simulink model "Full_Car_end_sem_Antiroll"  (R2023b)
settings: Solver=VariableStepAuto  StartTime=0.0  StopTime=20  FixedStep=0.00001  RelTol=1e-3
undefined symbols (not defined in the file): simscape, X, Y, Z
libraries: sm_lib x112, nesl_utility x70, fl_lib x23, sdl_lib x6, sharedtransform x4, simulink x2, simulink_extras x1
(part 6 of 6)

== system Full_Car_end_sem_Antiroll/Tire_RL/Tire_RL/Tire Visual ==
  Rigid Transform : sm_lib/Frames and Transforms/Rigid Transform  TranslationMethod=StandardAxis  TranslationStandardOffset=r0 - sectionHt/2  TranslationStandardOffsetUnits=m  TranslationStandardAxis=+Y  TranslationCartesianOffset=[0 0 0]  TranslationCartesianOffsetUnits=m  TranslationROffset=0  TranslationROffsetUnits=m  TranslationZOffset=0  TranslationZOffsetUnits=m  TranslationThetaOffset=0  TranslationThetaOffsetUnits=deg  RotationMethod=None  RotationAngleUnits=deg  RotationStandardAxis=+Z  RotationAngle=0.0  RotationArbitraryAxis=[0 0 1]  FollAlignAxisA=+X  BaseAlignAxisA=+Y  FollAlignAxisB=+Y  BaseAlignAxisB=+Z  RotationSequenceAxes=FollowerAxes  RotationSequence=XYX  RotationSequenceAngles=[0 0 0]  RotationSequenceAnglesUnits=deg  RotationMatrix=[1 0 0; 0 1 0; 0 0 1]  Quaternion=[1 0 0 0]
  Rigid Transform1 : sm_lib/Frames and Transforms/Rigid Transform  TranslationMethod=StandardAxis  TranslationStandardOffset=r0 - sectionHt/2  TranslationStandardOffsetUnits=m  TranslationStandardAxis=-Y  TranslationCartesianOffset=[0 0 0]  TranslationCartesianOffsetUnits=m  TranslationROffset=0  TranslationROffsetUnits=m  TranslationZOffset=0  TranslationZOffsetUnits=m  TranslationThetaOffset=0  TranslationThetaOffsetUnits=deg  RotationMethod=None  RotationAngleUnits=deg  RotationStandardAxis=+Z  RotationAngle=0.0  RotationArbitraryAxis=[0 0 1]  FollAlignAxisA=+X  BaseAlignAxisA=+Y  FollAlignAxisB=+Y  BaseAlignAxisB=+Z  RotationSequenceAxes=FollowerAxes  RotationSequence=XYX  RotationSequenceAngles=[0 0 0]  RotationSequenceAnglesUnits=deg  RotationMatrix=[1 0 0; 0 1 0; 0 0 1]  Quaternion=[1 0 0 0]
  Rigid Transform2 : sm_lib/Frames and Transforms/Rigid Transform  TranslationMethod=StandardAxis  TranslationStandardOffset=lr_val*(rimWidth/2-0.01)  TranslationStandardOffsetUnits=m  TranslationStandardAxis=+Z  TranslationCartesianOffset=[0 0 0]  TranslationCartesianOffsetUnits=m  TranslationROffset=0  TranslationROffsetUnits=m  TranslationZOffset=0  TranslationZOffsetUnits=m  TranslationThetaOffset=0  TranslationThetaOffsetUnits=deg  RotationMethod=None  RotationAngleUnits=deg  RotationStandardAxis=+Z  RotationAngle=0.0  RotationArbitraryAxis=[0 0 1]  FollAlignAxisA=+X  BaseAlignAxisA=+Y  FollAlignAxisB=+Y  BaseAlignAxisB=+Z  RotationSequenceAxes=FollowerAxes  RotationSequence=XYX  RotationSequenceAngles=[0 0 0]  RotationSequenceAnglesUnits=deg  RotationMatrix=[1 0 0; 0 1 0; 0 0 1]  Quaternion=[1 0 0 0]
  Rim : sm_lib/Body Elements/Extruded Solid  GraphicAmbientColor=[0.15 0.15 0.15 1.0]  BasedOnType=Density  CenterOfMass=[0 0 0]  CenterOfMassUnits=m  GraphicDiffuseColor=pulley_clr  ExportConvexHullGeometry=off  ExtrusionCrossSection=[x_rim',y_rim']  ExtrusionCrossSectionUnits=m  Density=0.001  DensityUnits=kg/m^3  DoExposeReferenceFrame=on  GraphicEmissiveColor=[0.0 0.0 0.0 1.0]  ExportEntireGeometry=off  ExtrusionLength=rimWidth  ExtrusionLengthUnits=m  ExtrusionType=General  SerializedFrames=<Frames/>  MarkerShape=Sphere  MarkerSize=10  GraphicType=FromGeometry  InertiaType=CalculateFromGeometry  Mass=1  MassUnits=kg  MomentsOfInertia=[1 1 1]  MomentsOfInertiaUnits=kg*m^2  PolygonNumSides=3  GraphicOpacity=pulley_opc  PolygonOuterRadius=1  PolygonOuterRadiusUnits=m  ProductsOfInertia=[0 0 0]  ProductsOfInertiaUnits=kg*m^2  GraphicShininess=75  GraphicSpecularColor=[0.5 0.5 0.5 1.0]  GraphicVisPropType=SimpleVisualProperties
  Rim design : sm_lib/Body Elements/Extruded Solid  GraphicAmbientColor=[0.15 0.15 0.15 1.0]  BasedOnType=Density  CenterOfMass=[0 0 0]  CenterOfMassUnits=m  GraphicDiffuseColor=pulley_clr  ExportConvexHullGeometry=off  ExtrusionCrossSection=[X,Y]  ExtrusionCrossSectionUnits=m  Density=0.001  DensityUnits=kg/m^3  DoExposeReferenceFrame=on  GraphicEmissiveColor=[0.0 0.0 0.0 1.0]  ExportEntireGeometry=off  ExtrusionLength=0.02  ExtrusionLengthUnits=m  ExtrusionType=General  SerializedFrames=<Frames/>  MarkerShape=Sphere  MarkerSize=10  GraphicType=FromGeometry  InertiaType=CalculateFromGeometry  Mass=1  MassUnits=kg  MomentsOfInertia=[1 1 1]  MomentsOfInertiaUnits=kg*m^2  PolygonNumSides=3  GraphicOpacity=pulley_opc  PolygonOuterRadius=1  PolygonOuterRadiusUnits=m  ProductsOfInertia=[0 0 0]  ProductsOfInertiaUnits=kg*m^2  GraphicShininess=75  GraphicSpecularColor=[0.5 0.5 0.5 1.0]  GraphicVisPropType=SimpleVisualProperties
  Tire : sm_lib/Body Elements/Extruded Solid  GraphicAmbientColor=[0.15 0.15 0.15 1.0]  BasedOnType=Density  CenterOfMass=[0 0 0]  CenterOfMassUnits=m  GraphicDiffuseColor=box_color  ExportConvexHullGeometry=off  ExtrusionCrossSection=[x_tire',y_tire']  ExtrusionCrossSectionUnits=m  Density=0.001  DensityUnits=kg/m^3  DoExposeReferenceFrame=on  GraphicEmissiveColor=[0.0 0.0 0.0 1.0]  ExportEntireGeometry=off  ExtrusionLength=rimWidth  ExtrusionLengthUnits=m  ExtrusionType=General  SerializedFrames=<Frames/>  MarkerShape=Sphere  MarkerSize=10  GraphicType=FromGeometry  InertiaType=CalculateFromGeometry  Mass=1  MassUnits=kg  MomentsOfInertia=[1 1 1]  MomentsOfInertiaUnits=kg*m^2  PolygonNumSides=3  GraphicOpacity=box_opc  PolygonOuterRadius=1  PolygonOuterRadiusUnits=m  ProductsOfInertia=[0 0 0]  ProductsOfInertiaUnits=kg*m^2  GraphicShininess=75  GraphicSpecularColor=[0.5 0.5 0.5 1.0]  GraphicVisPropType=SimpleVisualProperties
  C : PMIOPort  Side=Left
  connections:
  Rim design/RConn1 -- Rigid Transform2/RConn1
  Rigid Transform/RConn1 -- Rim/RConn1 -- Rigid Transform2/LConn1
  Rigid Transform/LConn1 -- Rigid Transform1/RConn1
  Rigid Transform1/LConn1 -- Tire/RConn1 -- C/RConn1

== system Full_Car_end_sem_Antiroll/Tire_RR/Tire_RR/Tire Visual ==
  Rigid Transform : sm_lib/Frames and Transforms/Rigid Transform  TranslationMethod=StandardAxis  TranslationStandardOffset=r0 - sectionHt/2  TranslationStandardOffsetUnits=m  TranslationStandardAxis=+Y  TranslationCartesianOffset=[0 0 0]  TranslationCartesianOffsetUnits=m  TranslationROffset=0  TranslationROffsetUnits=m  TranslationZOffset=0  TranslationZOffsetUnits=m  TranslationThetaOffset=0  TranslationThetaOffsetUnits=deg  RotationMethod=None  RotationAngleUnits=deg  RotationStandardAxis=+Z  RotationAngle=0.0  RotationArbitraryAxis=[0 0 1]  FollAlignAxisA=+X  BaseAlignAxisA=+Y  FollAlignAxisB=+Y  BaseAlignAxisB=+Z  RotationSequenceAxes=FollowerAxes  RotationSequence=XYX  RotationSequenceAngles=[0 0 0]  RotationSequenceAnglesUnits=deg  RotationMatrix=[1 0 0; 0 1 0; 0 0 1]  Quaternion=[1 0 0 0]
  Rigid Transform1 : sm_lib/Frames and Transforms/Rigid Transform  TranslationMethod=StandardAxis  TranslationStandardOffset=r0 - sectionHt/2  TranslationStandardOffsetUnits=m  TranslationStandardAxis=-Y  TranslationCartesianOffset=[0 0 0]  TranslationCartesianOffsetUnits=m  TranslationROffset=0  TranslationROffsetUnits=m  TranslationZOffset=0  TranslationZOffsetUnits=m  TranslationThetaOffset=0  TranslationThetaOffsetUnits=deg  RotationMethod=None  RotationAngleUnits=deg  RotationStandardAxis=+Z  RotationAngle=0.0  RotationArbitraryAxis=[0 0 1]  FollAlignAxisA=+X  BaseAlignAxisA=+Y  FollAlignAxisB=+Y  BaseAlignAxisB=+Z  RotationSequenceAxes=FollowerAxes  RotationSequence=XYX  RotationSequenceAngles=[0 0 0]  RotationSequenceAnglesUnits=deg  RotationMatrix=[1 0 0; 0 1 0; 0 0 1]  Quaternion=[1 0 0 0]
  Rigid Transform2 : sm_lib/Frames and Transforms/Rigid Transform  TranslationMethod=StandardAxis  TranslationStandardOffset=lr_val*(rimWidth/2-0.01)  TranslationStandardOffsetUnits=m  TranslationStandardAxis=+Z  TranslationCartesianOffset=[0 0 0]  TranslationCartesianOffsetUnits=m  TranslationROffset=0  TranslationROffsetUnits=m  TranslationZOffset=0  TranslationZOffsetUnits=m  TranslationThetaOffset=0  TranslationThetaOffsetUnits=deg  RotationMethod=None  RotationAngleUnits=deg  RotationStandardAxis=+Z  RotationAngle=0.0  RotationArbitraryAxis=[0 0 1]  FollAlignAxisA=+X  BaseAlignAxisA=+Y  FollAlignAxisB=+Y  BaseAlignAxisB=+Z  RotationSequenceAxes=FollowerAxes  RotationSequence=XYX  RotationSequenceAngles=[0 0 0]  RotationSequenceAnglesUnits=deg  RotationMatrix=[1 0 0; 0 1 0; 0 0 1]  Quaternion=[1 0 0 0]
  Rim : sm_lib/Body Elements/Extruded Solid  GraphicAmbientColor=[0.15 0.15 0.15 1.0]  BasedOnType=Density  CenterOfMass=[0 0 0]  CenterOfMassUnits=m  GraphicDiffuseColor=pulley_clr  ExportConvexHullGeometry=off  ExtrusionCrossSection=[x_rim',y_rim']  ExtrusionCrossSectionUnits=m  Density=0.001  DensityUnits=kg/m^3  DoExposeReferenceFrame=on  GraphicEmissiveColor=[0.0 0.0 0.0 1.0]  ExportEntireGeometry=off  ExtrusionLength=rimWidth  ExtrusionLengthUnits=m  ExtrusionType=General  SerializedFrames=<Frames/>  MarkerShape=Sphere  MarkerSize=10  GraphicType=FromGeometry  InertiaType=CalculateFromGeometry  Mass=1  MassUnits=kg  MomentsOfInertia=[1 1 1]  MomentsOfInertiaUnits=kg*m^2  PolygonNumSides=3  GraphicOpacity=pulley_opc  PolygonOuterRadius=1  PolygonOuterRadiusUnits=m  ProductsOfInertia=[0 0 0]  ProductsOfInertiaUnits=kg*m^2  GraphicShininess=75  GraphicSpecularColor=[0.5 0.5 0.5 1.0]  GraphicVisPropType=SimpleVisualProperties
  Rim design : sm_lib/Body Elements/Extruded Solid  GraphicAmbientColor=[0.15 0.15 0.15 1.0]  BasedOnType=Density  CenterOfMass=[0 0 0]  CenterOfMassUnits=m  GraphicDiffuseColor=pulley_clr  ExportConvexHullGeometry=off  ExtrusionCrossSection=[X,Y]  ExtrusionCrossSectionUnits=m  Density=0.001  DensityUnits=kg/m^3  DoExposeReferenceFrame=on  GraphicEmissiveColor=[0.0 0.0 0.0 1.0]  ExportEntireGeometry=off  ExtrusionLength=0.02  ExtrusionLengthUnits=m  ExtrusionType=General  SerializedFrames=<Frames/>  MarkerShape=Sphere  MarkerSize=10  GraphicType=FromGeometry  InertiaType=CalculateFromGeometry  Mass=1  MassUnits=kg  MomentsOfInertia=[1 1 1]  MomentsOfInertiaUnits=kg*m^2  PolygonNumSides=3  GraphicOpacity=pulley_opc  PolygonOuterRadius=1  PolygonOuterRadiusUnits=m  ProductsOfInertia=[0 0 0]  ProductsOfInertiaUnits=kg*m^2  GraphicShininess=75  GraphicSpecularColor=[0.5 0.5 0.5 1.0]  GraphicVisPropType=SimpleVisualProperties
  Tire : sm_lib/Body Elements/Extruded Solid  GraphicAmbientColor=[0.15 0.15 0.15 1.0]  BasedOnType=Density  CenterOfMass=[0 0 0]  CenterOfMassUnits=m  GraphicDiffuseColor=box_color  ExportConvexHullGeometry=off  ExtrusionCrossSection=[x_tire',y_tire']  ExtrusionCrossSectionUnits=m  Density=0.001  DensityUnits=kg/m^3  DoExposeReferenceFrame=on  GraphicEmissiveColor=[0.0 0.0 0.0 1.0]  ExportEntireGeometry=off  ExtrusionLength=rimWidth  ExtrusionLengthUnits=m  ExtrusionType=General  SerializedFrames=<Frames/>  MarkerShape=Sphere  MarkerSize=10  GraphicType=FromGeometry  InertiaType=CalculateFromGeometry  Mass=1  MassUnits=kg  MomentsOfInertia=[1 1 1]  MomentsOfInertiaUnits=kg*m^2  PolygonNumSides=3  GraphicOpacity=box_opc  PolygonOuterRadius=1  PolygonOuterRadiusUnits=m  ProductsOfInertia=[0 0 0]  ProductsOfInertiaUnits=kg*m^2  GraphicShininess=75  GraphicSpecularColor=[0.5 0.5 0.5 1.0]  GraphicVisPropType=SimpleVisualProperties
  C : PMIOPort  Side=Left
  connections:
  C/RConn1 -- Tire/RConn1 -- Rigid Transform1/LConn1
  Rigid Transform/LConn1 -- Rigid Transform1/RConn1
  Rigid Transform2/LConn1 -- Rim/RConn1 -- Rigid Transform/RConn1
  Rim design/RConn1 -- Rigid Transform2/RConn1

== system Full_Car_end_sem_Antiroll/6 DOF/Tx Sensor/non rotating follower - vehicle frame/AngAccl1 ==
  bx : Inport
  by : Inport  Port=2
  bz : Inport  Port=3
  bus creator4 : BusCreator  Inputs=3
  AngAccl : Outport
  wires:
  bx/1 -> bus creator4/1  "bx"
  by/1 -> bus creator4/2  "by"
  bz/1 -> bus creator4/3  "bz"
  bus creator4/1 -> AngAccl/1  "AngAcclVehFrame"

== system Full_Car_end_sem_Antiroll/6 DOF/Tx Sensor/non rotating follower - vehicle frame/Angvel1 ==
  wx : Inport
  wy : Inport  Port=2
  wz : Inport  Port=3
  bus creator4 : BusCreator  Inputs=3
  AngVel : Outport
  wires:
  bus creator4/1 -> AngVel/1  "AngVelVehFrame"
  wz/1 -> bus creator4/3  "wz"
  wy/1 -> bus creator4/2  "wy"
  wx/1 -> bus creator4/1  "wx"

== system Full_Car_end_sem_Antiroll/6 DOF/Tx Sensor/non rotating follower - vehicle frame/LinAccl1 ==
  ax : Inport
  ay : Inport  Port=2
  az : Inport  Port=3
  bus creator2 : BusCreator  Inputs=3
  LinAccl : Outport
  wires:
  bus creator2/1 -> LinAccl/1  "LinAcclVehFrame"
  az/1 -> bus creator2/3  "az"
  ax/1 -> bus creator2/1  "ax"
  ay/1 -> bus creator2/2  "ay"

== system Full_Car_end_sem_Antiroll/6 DOF/Tx Sensor/non rotating follower - vehicle frame/LinPos1 ==
  px : Inport
  py : Inport  Port=2
  pz : Inport  Port=3
  bus creator : BusCreator  Inputs=3
  LinPos : Outport
  wires:
  bus creator/1 -> LinPos/1  "LinPosVehFrame"
  px/1 -> bus creator/1  "px"
  pz/1 -> bus creator/3  "pz"
  py/1 -> bus creator/2  "py"

== system Full_Car_end_sem_Antiroll/6 DOF/Tx Sensor/non rotating follower - vehicle frame/LinVel1 ==
  vx : Inport
  vy : Inport  Port=2
  vz : Inport  Port=3
  bus creator1 : BusCreator  Inputs=3
  LinVel : Outport
  wires:
  vz/1 -> bus creator1/3  "vz"
  vy/1 -> bus creator1/2  "vy"
  vx/1 -> bus creator1/1  "vx"
  bus creator1/1 -> LinVel/1  "LinVelVehFrame"

== system Full_Car_end_sem_Antiroll/6 DOF/Tx Sensor/non rotating follower - vehicle frame/quaternion to angle1 ==
  q : Inport
  Quaternions to Rotation Angles : sharedtransform/Quaternions to Rotation Angles  rotationOrder=ZYX  aMode=aMode
  Selector : Selector  InputPortWidth=3  IndexOptions=Index vector (dialog)  Indices=3  OutputSizes=1
  Selector1 : Selector  InputPortWidth=3  IndexOptions=Index vector (dialog)  Indices=2  OutputSizes=1
  Selector2 : Selector  InputPortWidth=3  IndexOptions=Index vector (dialog)  Indices=1  OutputSizes=1
  bus creator3 : BusCreator  Inputs=3
  Ang : Outport
  wires:
  Quaternions to Rotation Angles/1 -> Selector1/1, Selector2/1, Selector/1
  Selector1/1 -> bus creator3/2  "ry"
  bus creator3/1 -> Ang/1  "AngVehFrame"
  Selector2/1 -> bus creator3/3  "rz"
  Selector/1 -> bus creator3/1  "rx"
  q/1 -> Quaternions to Rotation Angles/1

== system Full_Car_end_sem_Antiroll/6 DOF/Tx Sensor/world frame/AngAccl ==
  bx : Inport
  by : Inport  Port=2
  bz : Inport  Port=3
  bus creator4 : BusCreator  Inputs=3
  AngAccl : Outport
  wires:
  bus creator4/1 -> AngAccl/1  "AngAccl"
  bz/1 -> bus creator4/3  "bz"
  by/1 -> bus creator4/2  "by"
  bx/1 -> bus creator4/1  "bx"

== system Full_Car_end_sem_Antiroll/6 DOF/Tx Sensor/world frame/Angvel ==
  wx : Inport
  wy : Inport  Port=2
  wz : Inport  Port=3
  bus creator4 : BusCreator  Inputs=3
  AngVel : Outport
  wires:
  wx/1 -> bus creator4/1  "wx"
  wy/1 -> bus creator4/2  "wy"
  wz/1 -> bus creator4/3  "wz"
  bus creator4/1 -> AngVel/1  "AngVel"

== system Full_Car_end_sem_Antiroll/6 DOF/Tx Sensor/world frame/LinAccl ==
  ax : Inport
  ay : Inport  Port=2
  az : Inport  Port=3
  bus creator2 : BusCreator  Inputs=3
  LinAccl : Outport
  wires:
  ay/1 -> bus creator2/2  "ay"
  ax/1 -> bus creator2/1  "ax"
  az/1 -> bus creator2/3  "az"
  bus creator2/1 -> LinAccl/1  "LinAccl"

== system Full_Car_end_sem_Antiroll/6 DOF/Tx Sensor/world frame/LinPos ==
  px : Inport
  py : Inport  Port=2
  pz : Inport  Port=3
  bus creator : BusCreator  Inputs=3
  LinPos : Outport
  wires:
  py/1 -> bus creator/2  "py"
  pz/1 -> bus creator/3  "pz"
  px/1 -> bus creator/1  "px"
  bus creator/1 -> LinPos/1  "LinPos"

== system Full_Car_end_sem_Antiroll/6 DOF/Tx Sensor/world frame/LinVel ==
  vx : Inport
  vy : Inport  Port=2
  vz : Inport  Port=3
  bus creator1 : BusCreator  Inputs=3
  LinVel : Outport
  wires:
  bus creator1/1 -> LinVel/1  "LinVel"
  vx/1 -> bus creator1/1  "vx"
  vy/1 -> bus creator1/2  "vy"
  vz/1 -> bus creator1/3  "vz"

== system Full_Car_end_sem_Antiroll/6 DOF/Tx Sensor/world frame/quaternion to angle ==
  q : Inport
  Quaternions to Rotation Angles : sharedtransform/Quaternions to Rotation Angles  rotationOrder=ZYX  aMode=aMode
  Selector : Selector  InputPortWidth=3  IndexOptions=Index vector (dialog)  Indices=3  OutputSizes=1
  Selector1 : Selector  InputPortWidth=3  IndexOptions=Index vector (dialog)  Indices=2  OutputSizes=1
  Selector2 : Selector  InputPortWidth=3  IndexOptions=Index vector (dialog)  Indices=1  OutputSizes=1
  bus creator3 : BusCreator  Inputs=3
  Ang : Outport
  wires:
  q/1 -> Quaternions to Rotation Angles/1
  Selector/1 -> bus creator3/1  "rx"
  Selector2/1 -> bus creator3/3  "rz"
  bus creator3/1 -> Ang/1  "Ang"
  Selector1/1 -> bus creator3/2  "ry"
  Quaternions to Rotation Angles/1 -> Selector/1, Selector2/1, Selector1/1

== system Full_Car_end_sem_Antiroll/6DOF CG/Tx Sensor/non rotating follower - vehicle frame/AngAccl1 ==
  bx : Inport
  by : Inport  Port=2
  bz : Inport  Port=3
  bus creator4 : BusCreator  Inputs=3
  AngAccl : Outport
  wires:
  bx/1 -> bus creator4/1  "bx"
  by/1 -> bus creator4/2  "by"
  bz/1 -> bus creator4/3  "bz"
  bus creator4/1 -> AngAccl/1  "AngAcclVehFrame"

== system Full_Car_end_sem_Antiroll/6DOF CG/Tx Sensor/non rotating follower - vehicle frame/Angvel1 ==
  wx : Inport
  wy : Inport  Port=2
  wz : Inport  Port=3
  bus creator4 : BusCreator  Inputs=3
  AngVel : Outport
  wires:
  bus creator4/1 -> AngVel/1  "AngVelVehFrame"
  wz/1 -> bus creator4/3  "wz"
  wy/1 -> bus creator4/2  "wy"
  wx/1 -> bus creator4/1  "wx"

== system Full_Car_end_sem_Antiroll/6DOF CG/Tx Sensor/non rotating follower - vehicle frame/LinAccl1 ==
  ax : Inport
  ay : Inport  Port=2
  az : Inport  Port=3
  bus creator2 : BusCreator  Inputs=3
  LinAccl : Outport
  wires:
  bus creator2/1 -> LinAccl/1  "LinAcclVehFrame"
  az/1 -> bus creator2/3  "az"
  ax/1 -> bus creator2/1  "ax"
  ay/1 -> bus creator2/2  "ay"

== system Full_Car_end_sem_Antiroll/6DOF CG/Tx Sensor/non rotating follower - vehicle frame/LinPos1 ==
  px : Inport
  py : Inport  Port=2
  pz : Inport  Port=3
  bus creator : BusCreator  Inputs=3
  LinPos : Outport
  wires:
  bus creator/1 -> LinPos/1  "LinPosVehFrame"
  px/1 -> bus creator/1  "px"
  pz/1 -> bus creator/3  "pz"
  py/1 -> bus creator/2  "py"

== system Full_Car_end_sem_Antiroll/6DOF CG/Tx Sensor/non rotating follower - vehicle frame/LinVel1 ==
  vx : Inport
  vy : Inport  Port=2
  vz : Inport  Port=3
  bus creator1 : BusCreator  Inputs=3
  LinVel : Outport
  wires:
  vz/1 -> bus creator1/3  "vz"
  vy/1 -> bus creator1/2  "vy"
  vx/1 -> bus creator1/1  "vx"
  bus creator1/1 -> LinVel/1  "LinVelVehFrame"

== system Full_Car_end_sem_Antiroll/6DOF CG/Tx Sensor/non rotating follower - vehicle frame/quaternion to angle1 ==
  q : Inport
  Quaternions to Rotation Angles : sharedtransform/Quaternions to Rotation Angles  rotationOrder=ZYX  aMode=aMode
  Selector : Selector  InputPortWidth=3  IndexOptions=Index vector (dialog)  Indices=3  OutputSizes=1
  Selector1 : Selector  InputPortWidth=3  IndexOptions=Index vector (dialog)  Indices=2  OutputSizes=1
  Selector2 : Selector  InputPortWidth=3  IndexOptions=Index vector (dialog)  Indices=1  OutputSizes=1
  bus creator3 : BusCreator  Inputs=3
  Ang : Outport
  wires:
  Quaternions to Rotation Angles/1 -> Selector1/1, Selector2/1, Selector/1
  Selector1/1 -> bus creator3/2  "ry"
  bus creator3/1 -> Ang/1  "AngVehFrame"
  Selector2/1 -> bus creator3/3  "rz"
  Selector/1 -> bus creator3/1  "rx"
  q/1 -> Quaternions to Rotation Angles/1

== system Full_Car_end_sem_Antiroll/6DOF CG/Tx Sensor/world frame/AngAccl ==
  bx : Inport
  by : Inport  Port=2
  bz : Inport  Port=3
  bus creator4 : BusCreator  Inputs=3
  AngAccl : Outport
  wires:
  bus creator4/1 -> AngAccl/1  "AngAccl"
  bz/1 -> bus creator4/3  "bz"
  by/1 -> bus creator4/2  "by"
  bx/1 -> bus creator4/1  "bx"

== system Full_Car_end_sem_Antiroll/6DOF CG/Tx Sensor/world frame/Angvel ==
  wx : Inport
  wy : Inport  Port=2
  wz : Inport  Port=3
  bus creator4 : BusCreator  Inputs=3
  AngVel : Outport
  wires:
  wx/1 -> bus creator4/1  "wx"
  wy/1 -> bus creator4/2  "wy"
  wz/1 -> bus creator4/3  "wz"
  bus creator4/1 -> AngVel/1  "AngVel"

== system Full_Car_end_sem_Antiroll/6DOF CG/Tx Sensor/world frame/LinAccl ==
  ax : Inport
  ay : Inport  Port=2
  az : Inport  Port=3
  bus creator2 : BusCreator  Inputs=3
  LinAccl : Outport
  wires:
  ay/1 -> bus creator2/2  "ay"
  ax/1 -> bus creator2/1  "ax"
  az/1 -> bus creator2/3  "az"
  bus creator2/1 -> LinAccl/1  "LinAccl"

== system Full_Car_end_sem_Antiroll/6DOF CG/Tx Sensor/world frame/LinPos ==
  px : Inport
  py : Inport  Port=2
  pz : Inport  Port=3
  bus creator : BusCreator  Inputs=3
  LinPos : Outport
  wires:
  py/1 -> bus creator/2  "py"
  pz/1 -> bus creator/3  "pz"
  px/1 -> bus creator/1  "px"
  bus creator/1 -> LinPos/1  "LinPos"

== system Full_Car_end_sem_Antiroll/6DOF CG/Tx Sensor/world frame/LinVel ==
  vx : Inport
  vy : Inport  Port=2
  vz : Inport  Port=3
  bus creator1 : BusCreator  Inputs=3
  LinVel : Outport
  wires:
  bus creator1/1 -> LinVel/1  "LinVel"
  vx/1 -> bus creator1/1  "vx"
  vy/1 -> bus creator1/2  "vy"
  vz/1 -> bus creator1/3  "vz"

== system Full_Car_end_sem_Antiroll/6DOF CG/Tx Sensor/world frame/quaternion to angle ==
  q : Inport
  Quaternions to Rotation Angles : sharedtransform/Quaternions to Rotation Angles  rotationOrder=ZYX  aMode=aMode
  Selector : Selector  InputPortWidth=3  IndexOptions=Index vector (dialog)  Indices=3  OutputSizes=1
  Selector1 : Selector  InputPortWidth=3  IndexOptions=Index vector (dialog)  Indices=2  OutputSizes=1
  Selector2 : Selector  InputPortWidth=3  IndexOptions=Index vector (dialog)  Indices=1  OutputSizes=1
  bus creator3 : BusCreator  Inputs=3
  Ang : Outport
  wires:
  q/1 -> Quaternions to Rotation Angles/1
  Selector/1 -> bus creator3/1  "rx"
  Selector2/1 -> bus creator3/3  "rz"
  bus creator3/1 -> Ang/1  "Ang"
  Selector1/1 -> bus creator3/2  "ry"
  Quaternions to Rotation Angles/1 -> Selector/1, Selector2/1, Selector1/1
